simulink model "cruise_control_2024"  (R2024b)
settings: Solver=ode1  StartTime=0.0  StopTime=5  FixedStep=0.01  RelTol=1e-3
settings Model: Creator=Asus  LastModifiedBy=Asus
settings OptimizationCC: ZeroExternalMemoryAtStartup=off  ZeroInternalMemoryAtStartup=off
settings SFSimCC: SimUserSources=controller.cpp  SimTargetLang=C++
settings SFSimCC: SimCustomHeaderCode=|
  | extern "C" void compute_linear_model(int vehicle_id,
  |                           int road_id,
  |                           int weather_id,
  | 
  |                           double* K,
  |                           double* Tau,
  |                           double* Kp,
  |                           double* Ki,
  |                           double* Kd);
settings RTWCC: CustomHeaderCode=controller.h  CustomSource=controller.cpp  CustomInitializer=controller.cpp  TargetLang=C++
settings GRTTargetCC: TargetLangStandard=C++11 (ISO)  CodeInterfacePackaging=C++ class

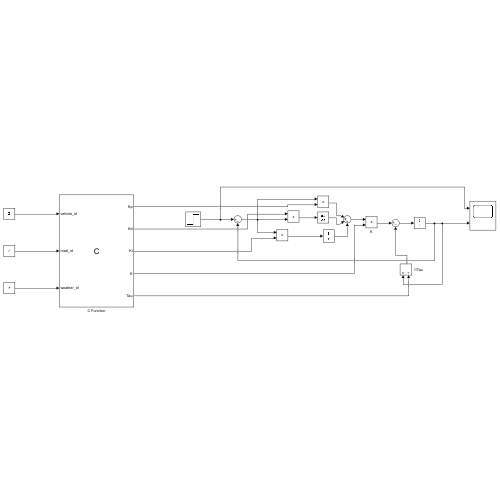
[thumbnail: Simulink's stored preview of the top-level diagram]
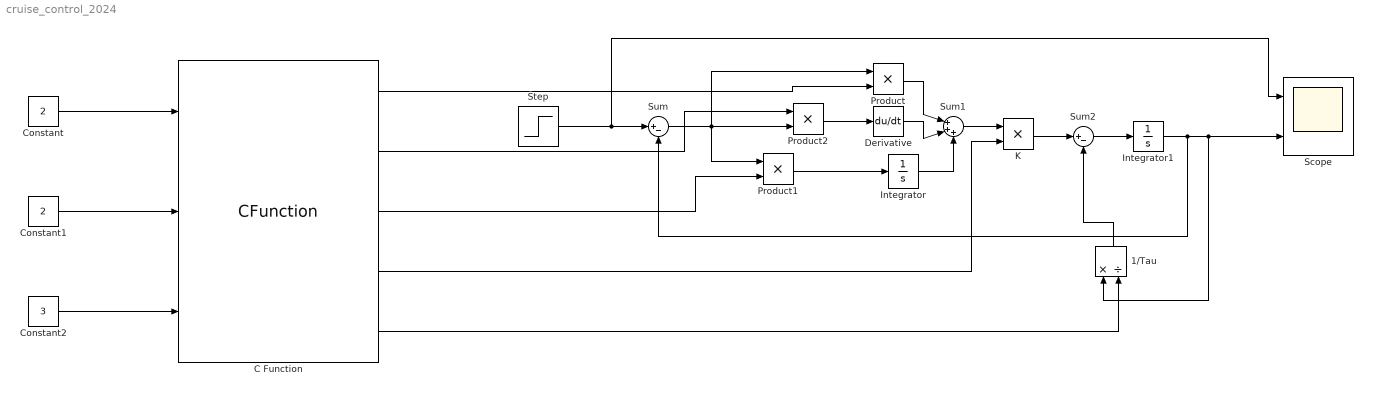
== system cruise_control_2024 ==
  1/Tau : Product  Inputs=*/
  C Function : CFunction  OutputCode=compute_linear_model( vehicle_id, road_id, weather_id, &K,&Tau,&Kp,&Ki,&Kd);  CodegenOutputCode=compute_linear_model( vehicle_id, road_id, weather_id, &K,&Tau,&Kp,&Ki,&Kd);  CustomCodeSettingLocation=ModelConfigurationParameters
  Constant : Constant  Value=2
  Constant1 : Constant  Value=2
  Constant2 : Constant  Value=3
  Derivative : Derivative
  Integrator : Integrator
  Integrator1 : Integrator
  K : Product
  Product : Product
  Product1 : Product
  Product2 : Product
  Scope : Scope  NumInputPorts=2
  Step : Step  After=100  SampleTime=0
  Sum : Sum  Inputs=|+-
  Sum1 : Sum  Inputs=|+++
  Sum2 : Sum  Inputs=|+-
  wires:
  Step/1 -> Sum/1, Scope/1
  Derivative/1 -> Sum1/2
  Product2/1 -> Derivative/1
  Product1/1 -> Integrator/1
  Integrator/1 -> Sum1/3
  Sum/1 -> Product2/2, Product1/1, Product/1
  C Function/1 -> Product/2
  Product/1 -> Sum1/1
  C Function/3 -> Product1/2
  C Function/2 -> Product2/1
  Sum1/1 -> K/1
  C Function/4 -> K/2
  K/1 -> Sum2/1
  Sum2/1 -> Integrator1/1
  Integrator1/1 -> 1/Tau/1, Scope/2, Sum/2
  1/Tau/1 -> Sum2/2
  C Function/5 -> 1/Tau/2
  Constant/1 -> C Function/1
  Constant1/1 -> C Function/2
  Constant2/1 -> C Function/3
